simulink model "test"  (Simulink 7.4)
settings: Solver=ode45  StartTime=0.0  StopTime=10.0  MaxStep=0.01  RelTol=1e-3
undefined symbols (not defined in the file or in its folder): sparse, x1, x2
libraries: BLOM_Lib x8
settings Model: Creator=JJK  LastModifiedBy=JJK
settings DebuggingCC: SolverPrmCheckMsg=none

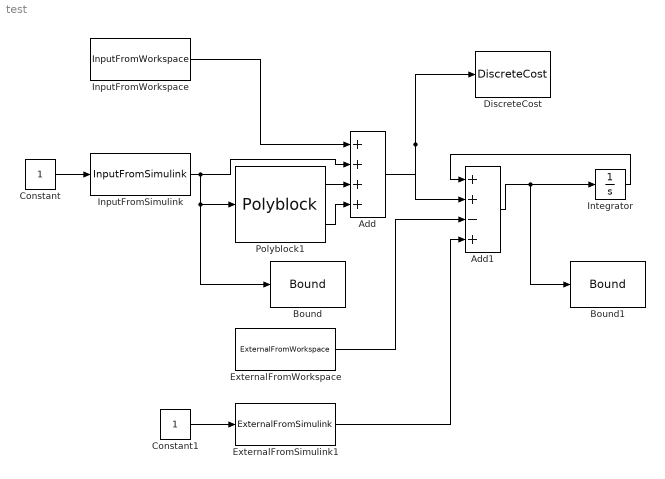
== system test ==
  Add : Sum  Inputs=++++  OutDataType=fixdt(1, 16)  OutScaling=2^-10
  Add1 : Sum  Inputs=++-+  OutDataType=fixdt(1, 16)  OutScaling=2^-10
  Bound : BLOM_Lib/Bound  SystemSampleTime=-1  ub=inf  lb=-inf  initial_step=on  final_step=on  intermediate_step=on
  Bound1 : BLOM_Lib/Bound  SystemSampleTime=-1  ub=inf  lb=-inf  initial_step=on  final_step=on  intermediate_step=on
  Constant : Constant  OutDataType=fixdt(1, 16)  OutScaling=2^0
  Constant1 : Constant  OutDataType=fixdt(1, 16)  OutScaling=2^0
  DiscreteCost : BLOM_Lib/DiscreteCost  SystemSampleTime=-1  initial_step=on  final_step=on  intermediate_step=on
  ExternalFromSimulink1 : BLOM_Lib/ExternalFromSimulink  SystemSampleTime=-1  interpType=Zero-Order Hold
  ExternalFromWorkspace : BLOM_Lib/ExternalFromWorkspace  SystemSampleTime=-1  simin=simin  interpType=Zero-Order Hold
  InputFromSimulink : BLOM_Lib/InputFromSimulink  SystemSampleTime=-1  interpType=Zero-Order Hold
  InputFromWorkspace : BLOM_Lib/InputFromWorkspace  SystemSampleTime=-1  simin=simin  interpType=Zero-Order Hold
  Integrator : Integrator
  Polyblock1 : BLOM_Lib/Polyblock  SystemSampleTime=-1  P=sparse([1 1 0; 3 1 0])  K=sparse([1 0.8; 1 1])  inputs=x1,x2  inputScalar=on  outputScalar=on
  wires:
  Constant/1 -> InputFromSimulink/1
  InputFromWorkspace/1 -> Add/1
  Add/1 -> DiscreteCost/1, Add1/2
  Integrator/1 -> Add1/1
  Add1/1 -> Integrator/1, Bound1/1
  ExternalFromWorkspace/1 -> Add1/3
  ExternalFromSimulink1/1 -> Add1/4
  Constant1/1 -> ExternalFromSimulink1/1
  Polyblock1/1 -> Add/3
  Polyblock1/2 -> Add/4
  InputFromSimulink/1 -> Add/2, Bound/1, Polyblock1/1
